simulink model "asig_directa_test"  (R2020b)
settings: Solver=FixedStepDiscrete  StartTime=0.0  StopTime=10.0  FixedStep=0.001  MaxStep=0.001  RelTol=1e-3
values from neighbouring files (symbols this model uses):
  AT = [0,                    1,                                   0, 0 ... (first row only)    [demo.m]    (also in pendulo_modelo.m)
  BT = [0;(M+m)*r*Kp/M/(J+r^2);0;-(M+m)*r*Kp/(J+r^2)/M/Lpend]    [demo.m]    (also in pendulo_modelo.m)
  C = [1, 0, 0, 0 ... (first row only)    [demo.m]    (also in pendulo_modelo.m)
  Gtd = c2d(Gt,T,'Tustin')    [demo.m]    (also in pendulo_modelo.m)
  Hd = place(Gtd.A',Gtd.C',pobsDiscrete)'    [demo.m]    (also in pendulo_modelo.m)
  K = place(Gt.A,Gt.B,pd)    [demo.m]    (also in pendulo_modelo.m)
  Kd = place(Gtd.A,Gtd.B,pDiscrete)    [demo.m]    (also in pendulo_modelo.m)
  Klqr = dlqr(Gtd.A,Gtd.B,Q,R)    [demo.m]    (also in pendulo_modelo.m)
  Robs = [1 0 ... (first row only)    [demo.m]    (also in pendulo_modelo.m)
undefined symbols (not defined in the file or in its folder): Discrete, Time
libraries: ctrlSharedLib x1
settings Model: Creator=aleca  LastModifiedBy=aleca

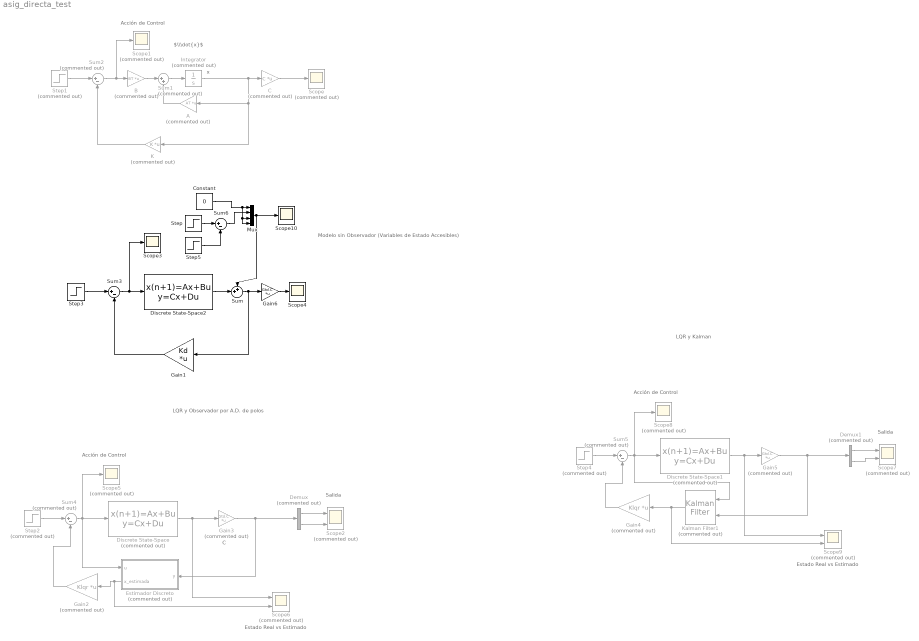
== system asig_directa_test ==
  note: Modelo sin Observador
      | (Variables de Estado Accesibles)
  note: C
  note: Acción de Control
  note: LQR y Kalman
  note: Acción de Control
  note: Salida
  note: Estado Real vs Estimado
  note: x
  note: $\\\dot{x}$
  note: Acción de Control
  note: Estado Real vs Estimado
  note: Salida
  note: LQR y Observador por A.D. de polos
  A : Gain  Commented=on  Gain=AT  Multiplication=Matrix(K*u)
  B : Gain  Commented=on  Gain=BT  Multiplication=Matrix(K*u)
  C : Gain  Commented=on  Gain=C  Multiplication=Matrix(K*u)
  Constant : Constant  Value=0
  Demux : Demux  Commented=on  Outputs=2
  Demux1 : Demux  Commented=on  Outputs=2
  Discrete State-Space : DiscreteStateSpace  Commented=on  A=Gtd.A  B=Gtd.B  C=eye(4)  D=zeros(4,1)  InitialCondition=[0 0 0 1]  SampleTime=-1
  Discrete State-Space1 : DiscreteStateSpace  Commented=on  A=Gtd.A  B=Gtd.B  C=eye(4)  D=zeros(4,1)  InitialCondition=[0 0 0.09 0.2]  SampleTime=-1
  Discrete State-Space2 : DiscreteStateSpace  A=Gtd.A  B=Gtd.B  C=eye(4)  D=zeros(4,1)  InitialCondition=[0.05 0 0.05 0]  SampleTime=-1
  Estimador Discreto : Subsystem  Commented=on
      settings: PortSchema="{\"entries\":[{\"content\":{\"sides\":[{\"content\":{\"connectorIds\":[\"In1\",\"Out1\"]},\"type\":\"ConnectorPlacement.EquallySpacedRectSide\",\"uuid\":\"54c951a6-c492-466a-87cc-2666df80341c\"},{\"content\":{\"connectorIds\":[\"In2\"],\"side\":\"RIGHT\"},\"type\":\"ConnectorPlacement.EquallySpacedRectSide\",\"uuid\":\"84d159db-5f82-478e-80b7-0aa3e5947a31\"},{\"content\":{\"connectorIds\":[],\"side\":\"TOP\"},\"type\":\"ConnectorPlacement.EquallySpacedRectSide\",\"uuid\":\"30ac016a-f884-45ce-a1da-2e3ef49bb594\"},{\"content\":{\"connectorIds\":[],\"side\":\"HIDDEN\"},\"type\":\"ConnectorPlacement.EquallySpacedRectSide\",\"uuid\":\"fc69af6f-3ea5-4985-ad9c-b3efd3bcb5d5\"}]},\"type\":\"ConnectorPlacement.EquallySpacedConnector\",\"uuid\":\"efc1973c-7238-45a0-b3a7-e4369d7e03c8\"}],\"packageUris\":[\"http://schema.mathworks.com/mf0/Connector/R2020b\"],\"version\":\"1.0\"}"
  Gain1 : Gain  Gain=Kd  Multiplication=Matrix(K*u)
  Gain2 : Gain  Commented=on  Gain=Klqr  Multiplication=Matrix(K*u)
  Gain3 : Gain  Commented=on  Gain=Gtd.C  Multiplication=Matrix(K*u)
  Gain4 : Gain  Commented=on  Gain=Klqr  Multiplication=Matrix(K*u)
  Gain5 : Gain  Commented=on  Gain=Gtd.C  Multiplication=Matrix(K*u)
  Gain6 : Gain  Gain=Gtd.C  Multiplication=Matrix(K*u)
  Integrator : Integrator  Commented=on
  K : Gain  Commented=on  Gain=K  Multiplication=Matrix(K*u)
  Kalman Filter1 : ctrlSharedLib/Kalman Filter  Commented=on  TimeDomain=Discrete-Time  UseCurrentEstimator=off  ModelSource=Individual A, B, C, D matrices  ModelSourceVariable=ss(0.95,1,1,0,1)  A=Gtd.A  B=Gtd.B  C=Gtd.C  D=Gtd.D  NumberOfStates=1  NumberOfInputs=1  NumberOfOutputs=1  InitialEstimateSource=Dialog  X0=0  P0=10  UseK=off  UseGH=off  NumberOfProcessNoiseInputs=1  G=1  TimeInvariantG=on  H=0  TimeInvariantH=on  Q=Qobs  TimeInvariantQ=on  R=Robs  TimeInvariantR=on  N=0  TimeInvariantN=on  AddInputPort=on  AddEnablePort=off  OutputEstimatedY=off  OutputP=off  Ts=-1
  Mux : Mux
  Scope{,1,5,8} (4 alike) : Scope  Commented=on
  Scope10 : Scope
  Scope{2,6..7,9} (4 alike) : Scope  Commented=on  NumInputPorts=2
  Scope3 : Scope
  Scope4 : Scope
  Step : Step  Time=4  After=0.5
  Step1 : Step  Commented=on  SampleTime=0
  Step2 : Step  Commented=on  After=0
  Step3 : Step  After=0  SampleTime=0
  Step4 : Step  Commented=on  After=0
  Step5 : Step  Time=4.01  After=0.5
  Sum : Sum  Inputs=++|
  Sum1 : Sum  Commented=on  Inputs=|++
  Sum2 : Sum  Commented=on  Inputs=|+-
  Sum3 : Sum  Inputs=|+-
  Sum4 : Sum  Commented=on  Inputs=|+-
  Sum5 : Sum  Commented=on  Inputs=|+-
  Sum6 : Sum  Inputs=|+-
  wires:
  B/1 -> Sum1/1
  Sum1/1 -> Integrator/1
  A/1 -> Sum1/2
  C/1 -> Scope/1
  Sum2/1 -> Scope1/1, B/1
  Step1/1 -> Sum2/1
  K/1 -> Sum2/2
  Integrator/1 -> K/1, A/1, C/1
  Step3/1 -> Sum3/1
  Gain1/1 -> Sum3/2
  Sum3/1 -> Discrete State-Space2/1, Scope3/1
  Step2/1 -> Sum4/1
  Sum4/1 -> Estimador Discreto/1(u), Discrete State-Space/1, Scope5/1
  Gain2/1 -> Sum4/2
  Gain3/1 -> Estimador Discreto/2(y), Demux/1
  Discrete State-Space/1 -> Scope6/1, Gain3/1
  Demux/1 -> Scope2/1
  Demux/2 -> Scope2/2
  Demux1/2 -> Scope7/2
  Demux1/1 -> Scope7/1
  Gain4/1 -> Sum5/2
  Gain5/1 -> Kalman Filter1/2, Demux1/1
  Discrete State-Space1/1 -> Scope9/1, Gain5/1
  Step4/1 -> Sum5/1
  Sum5/1 -> Kalman Filter1/1, Discrete State-Space1/1, Scope8/1
  Kalman Filter1/1 -> Scope9/2, Gain4/1
  Estimador Discreto/1(x_estimada) -> Scope6/2, Gain2/1
  Gain6/1 -> Scope4/1
  Sum/1 -> Gain6/1, Gain1/1
  Discrete State-Space2/1 -> Sum/2
  Constant/1 -> Mux/4, Mux/3, Mux/1
  Mux/1 -> Sum/1, Scope10/1
  Step/1 -> Sum6/1
  Step5/1 -> Sum6/2
  Sum6/1 -> Mux/2

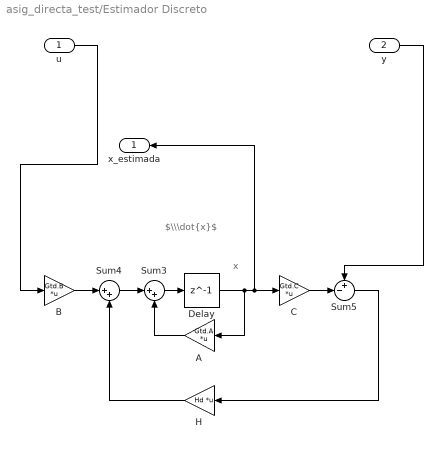
== system asig_directa_test/Estimador Discreto ==
  note: $\\\dot{x}$
  note: x
  u : Inport
  y : Inport  Port=2
  A : Gain  Gain=Gtd.A  Multiplication=Matrix(K*u)
  B : Gain  Gain=Gtd.B  Multiplication=Matrix(K*u)
  C : Gain  Gain=Gtd.C  Multiplication=Matrix(K*u)
  Delay : Delay  DelayLength=1
  H : Gain  Gain=Hd  Multiplication=Matrix(K*u)
  Sum3 : Sum  Inputs=|++
  Sum4 : Sum  Inputs=|++
  Sum5 : Sum  Inputs=+-|
  x_estimada : Outport
  wires:
  B/1 -> Sum4/1
  Delay/1 -> x_estimada/1, C/1, A/1
  Sum3/1 -> Delay/1
  y/1 -> Sum5/1
  Sum4/1 -> Sum3/1
  H/1 -> Sum4/2
  C/1 -> Sum5/2
  A/1 -> Sum3/2
  Sum5/1 -> H/1
  u/1 -> B/1
